simulink model "testthrustmdl"  (Simulink 7.7)
settings: Solver=ode45  StartTime=0.0  StopTime=5  RelTol=1e-3
settings Model: Creator=Administrator  LastModifiedBy=Administrator
settings DataIOCC: OutputSaveName=T_MR

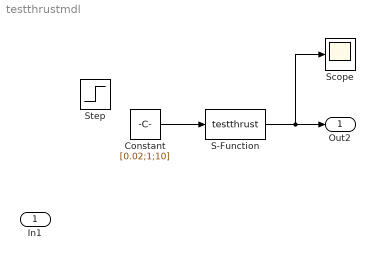
== system testthrustmdl ==
  In1 : Inport
  Constant : Constant  Value=[0.02;1;10]
  S-Function : S-Function  FunctionName=testthrust  EnableBusSupport=off
  Scope : Scope
  Step : Step  Time=0  After=0  SampleTime=0
  Out2 : Outport
  wires:
  S-Function/1 -> Out2/1, Scope/1
  Constant/1 -> S-Function/1
